simulink model "estTest"  (R2021b)
settings: Solver=FixedStepAuto  StartTime=0.0  StopTime=600  RelTol=1e-3
StartFcn:
  | hardwareSetup;
model workspace (MAT data in the model file):
  Ts = Simulink.Parameter
  Ts.Value = 0.005
  Ts.DataType = 'auto'
  Ts.Complexity = 'real'
  Ts.Dimensions = [1 1]
  stepH = Simulink.Parameter
  stepH.Value = 60
  stepH.DataType = 'auto'
  stepH.Complexity = 'real'
  stepH.Dimensions = [1 1]
  stepL = Simulink.Parameter
  stepL.Value = 50
  stepL.DataType = 'auto'
  stepL.Complexity = 'real'
  stepL.Dimensions = [1 1]
  tF = Simulink.Parameter
  tF.Value = 0.3
  tF.DataType = 'auto'
  tF.Complexity = 'real'
  tF.Dimensions = [1 1]
  tS = Simulink.Parameter
  tS.Value = 0.3
  tS.DataType = 'auto'
  tS.Complexity = 'real'
  tS.Dimensions = [1 1]
values from neighbouring files (symbols this model uses):
  Ts = 0.025    [MPCGen_OffsetFree.m]    (also in MPCGen_OffsetFree_UD.m = 0.02; MPCGen_OffsetFree_estDis.m = 0.03; MPCcontrollerGen_OffsetFree.m; MPCcontrollerGen_OffsetFree_UD.m = 0.02)
libraries: PuppyLibrary x6
settings Model: SimulationMode=external  ExtModeTrigDuration=2  Creator=kboxi  LastModifiedBy=MSI-NB
settings SolverCC: AlgebraicLoopSolver=TrustRegion  PositivePriorityOrder=on
settings DataIOCC: LimitDataPoints=on  MaxDataPoints=10000
settings OptimizationCC: DefaultParameterBehavior=Inlined  MaxStackSize=64
settings DebuggingCC: ParameterTunabilityLossMsg=error  SFMachineParentedDataDiag=warning  ArithmeticOperatorsInVariantConditions=warning
settings HardwareCC: ProdBitPerPointer=32  ProdBitPerSizeT=32  ProdBitPerPtrDiffT=32  ProdLargestAtomicInteger=Long  ProdLargestAtomicFloat=Double  ProdWordSize=32  ProdHWDeviceType=ARM Compatible->ARM Cortex  UseEmbeddedCoderFeatures=off
settings SFSimCC: SimUseLocalCustomCode=off  CustomCodeUndefinedFunction=UseInterfaceOnly
settings RTWCC: Description=Embedded Coder  SystemTargetFile=ert.tlc  HardwareBoard=Raspberry Pi  TLCOptions="-aInlineSetEventsForThisBaseRateFcn=TLC_FALSE -aSuppressMultiTaskScheduler=TLC_FALSE  -aRateBasedStepFcn=0"  TemplateMakefile=ert_default_tmf  RTWUseLocalCustomCode=off  Toolchain=GNU GCC Embedded Linux  BuildConfiguration=Faster Runs
settings CodeAppCC: ForceParamTrailComments=on  GenerateComments=off  OperatorAnnotations=on  StateflowObjectComments=on  MATLABSourceComments=on
settings ERTTargetCC: ERTCustomFileBanners=off  MatFileLogging=on  SupportContinuousTime=on  SupportNonInlinedSFcns=on  RemoveResetFunc=off  SupportVariableSizeSignals=on  ModelStepFunctionPrototypeControlCompliant=off  ExtModeTransport=2  ExtModeStaticAlloc=on  ExtModeMexFile=ext_xcp  ExtModeIntrfLevel=Level2 - Open

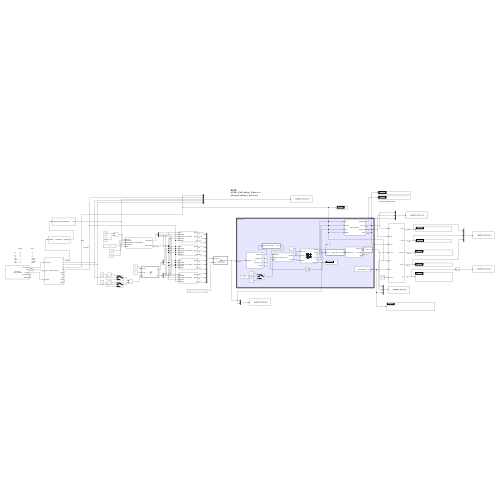
[thumbnail: Simulink's stored preview of the top-level diagram]
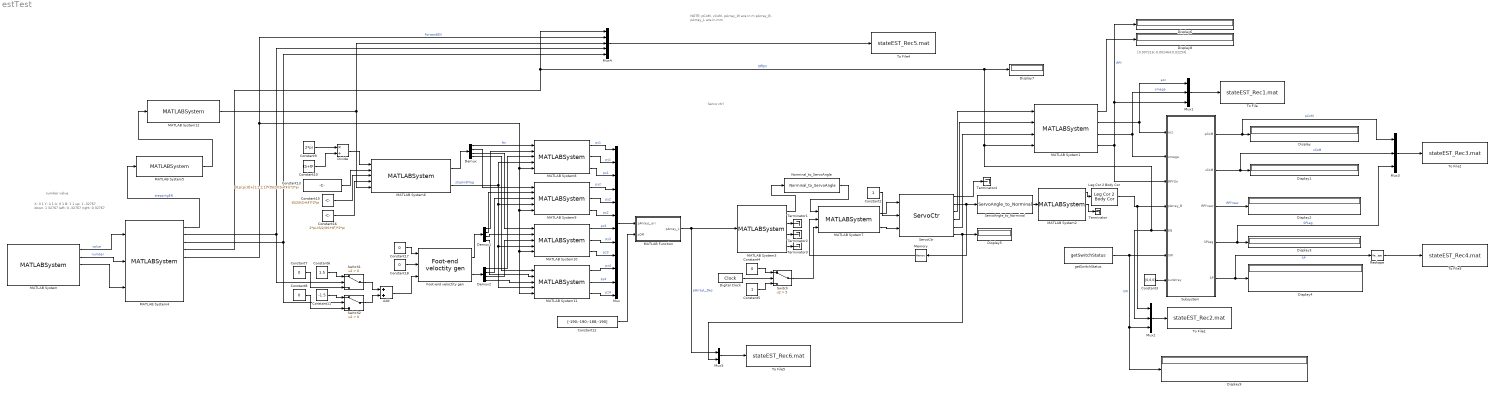
== system estTest ==
  note: NOTE:
      | pCoM, vCoM, pArray_W are in m
      | pArray_B, pArray_L are in mm
  note: Servo ctrl
  note: number value
  note: X:            3                                   1
      | Y:            4                                   1
      | A:            0                                   1
      | B:            1                                   1
      | up:           1                               -32767
      | down:      1                                32767
      | left:          0                                -32767
      | right:        0                               32767
  note: [0.007216;-0.002464;0.02254]
  Add : Sum
  Constant10 : Constant  Value=tS+tF
  Constant11 : Constant  Value=-1.5
  Constant12 : Constant  Value=[-190;-190;-188;-190]
  Constant13 : Constant  Value=[0;pi;pi;0]+[1;1;1;1]*(tS/2/(tS+tF))*2*pi
  Constant15 : Constant  Value=tS/2/(tS+tF)*2*pi
  Constant16 : Constant  Value=2*pi-tS/2/(tS+tF)*2*pi
  Constant{4,7..8,17..18} (5 alike) : Constant  Value=0
  Constant2 : Constant
  Constant3 : Constant  Value=[0,0,0]
  Constant5 : Constant
  Constant6 : Constant  Value=1.5
  Constant9 : Constant  Value=2*pi
  Demux : Demux
  Demux1 : Demux
  Demux2 : Demux
  Digital Clock : DigitalClock  SampleTime=Ts
  Display{,1..9} (10 alike) : Display
  Divide : Product  Inputs=*/
  Foot-end veloctity gen : PuppyLibrary/Foot-end veloctity gen  SystemSampleTime=-1  VariantActivationTime=update diagram  Latency=0  AutoFrameSizeCalculation=off
  Leg Cor 2 Body Cor : PuppyLibrary/Leg Cor 2 Body Cor  SystemSampleTime=-1  VariantActivationTime=update diagram  Latency=0  AutoFrameSizeCalculation=off
  MATLAB Function : MATLAB Function  TreatAsAtomicUnit=on
  MATLAB System : MATLABSystem  System=JoystickRead  SampleTime=0.005
      mask Type: JoystickRead
      mask Display:
      | disp(['Bluetooth' char(10) ' Joystick Reader']);
      | port_label('output',1,'EventNum');
      | port_label('output',2,'value');
      | port_label('output',3,'number');
      | port_label('output',4,'buttonState');
      | port_label('output',5,'axisState');
  MATLAB System1 : MATLABSystem  System=IMU_regulation  SimulateUsing=Code generation
      mask Type: IMU_regulation
      mask Display:
      | disp('IMU_regulation');
      | port_label('input',1,'acc');
      | port_label('input',2,'omega');
      | port_label('input',3,'rpy');
      | port_label('input',4,'OffEN');
      | port_label('output',1,'accOffnow');
      | port_label('output',2,'accL_W');
      | port_label('output',3,'omega_W');
      | port_label('output',4,'RPY');
  MATLAB System10 : MATLABSystem  System=cycCurveGen  Tf=tF  Ts=tS  H=stepH  L=stepL  Hsd=3  dt=Ts  SimulateUsing=Code generation
      mask Type: cycCurveGen
      mask Display:
      | disp('cycCurveGen');
      | port_label('input',1,'fai');
      | port_label('input',2,'vpxAdd');
      | port_label('input',3,'vpyAdd');
      | port_label('input',4,'stopInd');
      | port_label('input',5,'xADes');
      | port_label('output',1,'pxOut');
      | port_label('output',2,'pyOut');
      | port_label('output',3,'pz');
  MATLAB System11 : MATLABSystem  System=cycCurveGen  Tf=tF  Ts=tS  H=stepH  L=stepL  Hsd=4  dt=Ts  SimulateUsing=Code generation
      mask Type: cycCurveGen
      mask Display:
      | disp('cycCurveGen');
      | port_label('input',1,'fai');
      | port_label('input',2,'vpxAdd');
      | port_label('input',3,'vpyAdd');
      | port_label('input',4,'stopInd');
      | port_label('input',5,'xADes');
      | port_label('output',1,'pxOut');
      | port_label('output',2,'pyOut');
      | port_label('output',3,'pz');
  MATLAB System12 : MATLABSystem  System=ButtonHoldviaEdge  SimulateUsing=Code generation
      mask Type: ButtonHoldviaEdge
      mask Display:
      | disp('ButtonHoldviaEdge');
      | port_label('input',1,'dataEdge');
      | port_label('output',1,'data');
  MATLAB System2 : MATLABSystem  System=FK  dt=0.005  SimulateUsing=Code generation
      mask Type: FK
      mask Display:
      | disp('FK');
      | port_label('input',1,'AngleArray');
      | port_label('output',1,'pArray_L');
      | port_label('output',2,'errFlag');
      | port_label('output',3,'dq');
  MATLAB System3 : MATLABSystem  System=IK  LF_Off=[ 0; 0; 0 ]  RF_Off=[ 0; 0; 0 ]  LH_Off=[ 0; 0; 0 ]  RH_Off=[ 0; 0; 0 ]  SimulateUsing=Code generation
      mask Type: IK
      mask Display:
      | disp('IK');
      | port_label('input',1,'pArray_L');
      | port_label('output',1,'AngleArray');
      | port_label('output',2,'OffsetPArray');
      | port_label('output',3,'pArray_L_Out');
      | port_label('output',4,'errFlag');
  MATLAB System4 : MATLABSystem  System=buttonDecoder_2  SimulateUsing=Code generation
      mask Type: buttonDecoder_2
      mask Display:
      | disp('buttonDecoder_2');
      | port_label('input',1,'Eventnum');
      | port_label('input',2,'value');
      | port_label('input',3,'number');
      | port_label('output',1,'X');
      | port_label('output',2,'Y');
      | port_label('output',3,'A');
      | port_label('output',4,'B');
      | port_label('output',5,'up');
      | port_label('output',6,'down');
      | port_label('output',7,'left');
      | port_label('output',8,'right');
      | port_label('output',9,'LAxis');
      | port_label('output',10,'RAxis');
  MATLAB System5 : MATLABSystem  System=edgeDetector  SimulateUsing=Code generation
      mask Type: edgeDetector
      mask Display:
      | disp('edgeDetector');
      | port_label('input',1,'dataNow');
      | port_label('output',1,'dataEdge');
  MATLAB System6 : MATLABSystem  System=PhaseOscillator  SampleTime=Ts  OffsetTime=0  TickTime=0.1  SimulateUsing=Code generation
      mask Type: PhaseOscillator
      mask Display:
      | disp('PhaseOscillator');
      | port_label('input',1,'omega');
      | port_label('input',2,'phaseLag');
      | port_label('input',3,'stopIndPhase');
      | port_label('input',4,'stopPhase');
      | port_label('input',5,'EN');
      | port_label('output',1,'phaseNow');
      | port_label('output',2,'stopIndFlag');
  MATLAB System7 : MATLABSystem  System=PosAssign_vel  cons_Vel=15  dt=Ts  SimulateUsing=Code generation
      mask Type: PosAssign_vel
      mask Display:
      | disp('PosAssign_vel');
      | port_label('input',1,'PosDes');
      | port_label('input',2,'PosNow');
      | port_label('input',3,'EN');
      | port_label('output',1,'PosOut');
      | port_label('output',2,'setEN');
  MATLAB System8 : MATLABSystem  System=cycCurveGen  Tf=tF  Ts=tS  H=stepH  L=stepL  Hsd=4  dt=Ts  SimulateUsing=Code generation
      mask Type: cycCurveGen
      mask Display:
      | disp('cycCurveGen');
      | port_label('input',1,'fai');
      | port_label('input',2,'vpxAdd');
      | port_label('input',3,'vpyAdd');
      | port_label('input',4,'stopInd');
      | port_label('input',5,'xADes');
      | port_label('output',1,'pxOut');
      | port_label('output',2,'pyOut');
      | port_label('output',3,'pz');
  MATLAB System9 : MATLABSystem  System=cycCurveGen  Tf=tF  Ts=tS  H=stepH  L=stepL  Hsd=4  dt=Ts  SimulateUsing=Code generation
      mask Type: cycCurveGen
      mask Display:
      | disp('cycCurveGen');
      | port_label('input',1,'fai');
      | port_label('input',2,'vpxAdd');
      | port_label('input',3,'vpyAdd');
      | port_label('input',4,'stopInd');
      | port_label('input',5,'xADes');
      | port_label('output',1,'pxOut');
      | port_label('output',2,'pyOut');
      | port_label('output',3,'pz');
  Memory : Memory  InitialCondition=zeros(12,1)
  Mux : Mux  Inputs=12
  Mux1 : Mux  Inputs=3
  Mux2 : Mux  Inputs=3
  Mux3 : Mux  Inputs=3
  Mux4 : Mux  Inputs=5
  Mux5 : Mux  Inputs=2
  Norminal_to_ServoAngle : PuppyLibrary/Norminal_to_ServoAngle  SystemSampleTime=-1  VariantActivationTime=update diagram  Latency=0  AutoFrameSizeCalculation=off
  Reshape : Reshape
  ServoAngle_to_Norminal : PuppyLibrary/ServoAngle_to_Norminal  SystemSampleTime=-1  VariantActivationTime=update diagram  Latency=0  AutoFrameSizeCalculation=off
  ServoCtr : PuppyLibrary/ServoCtr  SystemSampleTime=-1  VariantActivationTime=update diagram  Latency=0  AutoFrameSizeCalculation=off
  Subsystem : Subsystem
  Switch : Switch  Criteria=u2 > Threshold  Threshold=5
  Switch1 : Switch  Criteria=u2 > Threshold
  Switch2 : Switch  Criteria=u2 > Threshold
  Terminator{,1..4} (5 alike) : Terminator
  To File : ToFile  Filename=stateEST_Rec1.mat  MatrixName=in_acc_omega_RPY
  To File1 : ToFile  Filename=stateEST_Rec2.mat  MatrixName=in_pArrayB_EN_SW
  To File2 : ToFile  Filename=stateEST_Rec3.mat  MatrixName=est_pCoM_vCoM_SPLeg
  To File3 : ToFile  Filename=stateEST_Rec4.mat  MatrixName=est_SP
  To File4 : ToFile  Filename=stateEST_Rec5.mat  MatrixName=est_offEN_forward_step_left_right
  To File5 : ToFile  Filename=stateEST_Rec6.mat  MatrixName=est_pArrayLDes_stm32Error
  getSwitchStatus : PuppyLibrary/getSwitchStatus  sampleTime=0.005
  wires:
  Reshape/1 -> To File3/1
  MATLAB System4/3 -> Switch2/2, Mux4/5
  MATLAB System4/4 -> Mux4/1, Mux2/2, Subsystem/5(EN), MATLAB System1/4, Display7/1  "OffEN"
  MATLAB System5/1 -> MATLAB System12/1
  Mux1/1 -> To File/1
  Mux2/1 -> To File1/1
  MATLAB System2/1 -> Leg Cor 2 Body Cor/1
  MATLAB System4/5 -> Mux4/2, MATLAB System8/5, MATLAB System11/5, MATLAB System10/5, MATLAB System9/5  "ForwardEN"
  MATLAB System2/2 -> Terminator/1
  MATLAB System1/3 -> Mux1/2, Subsystem/2(omega)  "omega"
  MATLAB System1/2 -> Subsystem/1(acc), Mux1/1  "acc"
  MATLAB System9/3 -> Mux/6  "pz2"
  MATLAB System1/4 -> Mux1/3, Display6/1, Subsystem/3(RPYOri)  "RPY"
  Demux1/1 -> MATLAB System8/2
  ServoCtr/4 -> MATLAB System1/2
  MATLAB System8/2 -> Mux/2  "py1"
  MATLAB System4/2 -> Switch1/2, Mux4/4
  Demux2/4 -> MATLAB System11/3
  MATLAB System3/3 -> Terminator2/1
  ServoCtr/1 -> Terminator4/1
  getSwitchStatus/1 -> Display9/1, Mux2/3, Subsystem/6(SW)  "SW"
  Memory/1 -> MATLAB System7/2
  MATLAB System6/2 -> MATLAB System11/4, MATLAB System10/4, MATLAB System9/4, MATLAB System8/4  "stopIndFlag"
  MATLAB System1/1 -> Display8/1
  Constant6/1 -> Switch1/1
  Switch2/1 -> Add/2
  Constant13/1 -> MATLAB System6/2
  Demux/2 -> MATLAB System9/1
  MATLAB System7/2 -> ServoCtr/3
  ServoCtr/6 -> Mux5/2, Display5/1
  ServoCtr/3 -> MATLAB System1/1
  MATLAB System11/3 -> Mux/12  "pz4"
  MATLAB Function/1(pArray_L) -> Mux5/1, MATLAB System3/1  "pArrayL_Des"
  ServoCtr/5 -> MATLAB System1/3
  MATLAB System8/1 -> Mux/1  "px1"
  MATLAB System/3 -> MATLAB System4/3
  Subsystem/5(SP) -> Reshape/1, Display4/1  "SP"
  Demux2/1 -> MATLAB System8/3
  Constant12/1 -> MATLAB Function/2(zOff)
  Mux/1 -> MATLAB Function/1(pArrayL_ori)
  Constant7/1 -> Switch1/3
  Demux/3 -> MATLAB System10/1
  Subsystem/1(pCoM) -> Mux3/1, Display/1  "pCoM"
  Switch1/1 -> Add/1
  MATLAB System11/2 -> Mux/11  "py4"
  Demux2/3 -> MATLAB System10/3
  Constant8/1 -> Switch2/3
  MATLAB System12/1 -> Mux4/3, MATLAB System6/5
  Demux1/4 -> MATLAB System11/2
  MATLAB System3/1 -> Norminal_to_ServoAngle/1
  MATLAB System10/3 -> Mux/9  "pz3"
  MATLAB System11/1 -> Mux/10  "px4"
  Add/1 -> Foot-end veloctity gen/3
  MATLAB System9/2 -> Mux/5  "py2"
  ServoCtr/2 -> Memory/1, ServoAngle_to_Norminal/1
  MATLAB System3/4 -> Terminator3/1
  Constant17/1 -> Foot-end veloctity gen/1
  Foot-end veloctity gen/1 -> Demux1/1
  Constant9/1 -> Divide/1
  Divide/1 -> MATLAB System6/1
  Foot-end veloctity gen/2 -> Demux2/1
  MATLAB System6/1 -> Demux/1
  Norminal_to_ServoAngle/1 -> MATLAB System7/1
  Constant16/1 -> MATLAB System6/4
  MATLAB System8/3 -> Mux/3  "pz1"
  Constant4/1 -> Switch/1
  Demux/4 -> MATLAB System11/1
  Digital Clock/1 -> Switch/2
  Constant15/1 -> MATLAB System6/3
  Demux1/2 -> MATLAB System9/2
  ServoAngle_to_Norminal/1 -> MATLAB System2/1
  Subsystem/4(SPLeg) -> Mux3/3, Display3/1  "SPLeg"
  MATLAB System10/2 -> Mux/8  "py3"
  Demux2/2 -> MATLAB System9/3
  Constant18/1 -> Foot-end veloctity gen/2
  Subsystem/3(RPYnew) -> Display2/1  "RPYnew"
  Constant5/1 -> Switch/3
  Constant3/1 -> Subsystem/7(surArray)
  MATLAB System4/1 -> MATLAB System5/1  "steppingEN"
  Constant2/1 -> ServoCtr/2
  Switch/1 -> MATLAB System7/3
  MATLAB System10/1 -> Mux/7  "px3"
  MATLAB System3/2 -> Terminator1/1
  Constant11/1 -> Switch2/1
  MATLAB System9/1 -> Mux/4  "px2"
  MATLAB System/2 -> MATLAB System4/2  "number"
  Demux/1 -> MATLAB System8/1  "fai"
  Leg Cor 2 Body Cor/1 -> Mux2/1, Subsystem/4(pArray_B)
  Demux1/3 -> MATLAB System10/2
  Mux3/1 -> To File2/1
  MATLAB System7/1 -> ServoCtr/1
  Subsystem/2(vCoM) -> Mux3/2, Display1/1  "vCoM"
  MATLAB System/1 -> MATLAB System4/1  "value"
  Constant10/1 -> Divide/2
  Mux4/1 -> To File4/1
  Mux5/1 -> To File5/1

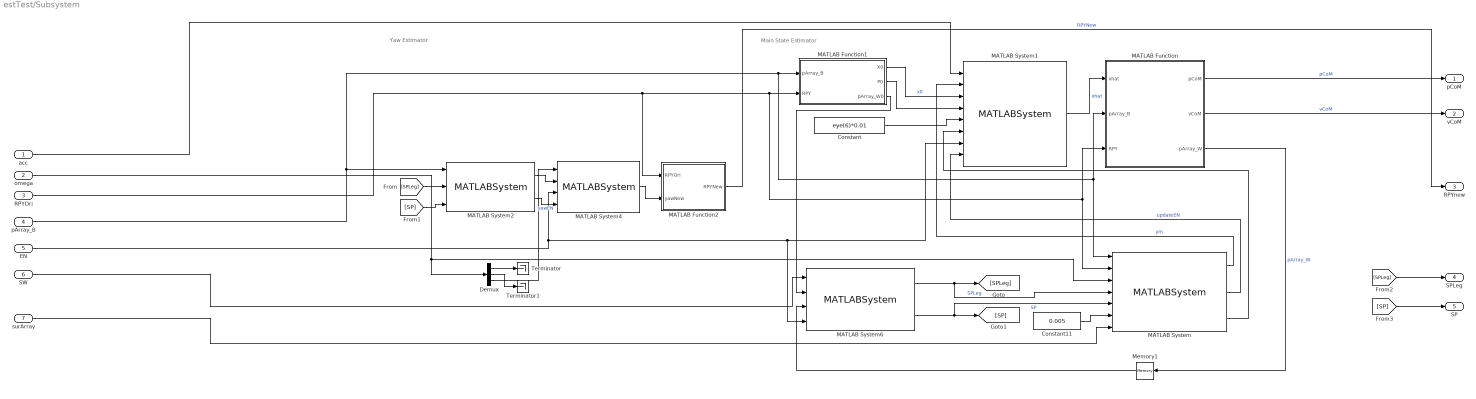
== system estTest/Subsystem ==
  note: Yaw Estimator
  note: Main State Estimator
  acc : Inport
  omega : Inport  Port=2
  RPYOri : Inport  Port=3
  pArray_B : Inport  Port=4
  EN : Inport  Port=5
  SW : Inport  Port=6
  surArray : Inport  Port=7
  Constant : Constant  Value=eye(6)*0.01
  Constant11 : Constant  Value=0.005
  Demux : Demux  Outputs=3
  MATLAB Function : MATLAB Function  TreatAsAtomicUnit=on
  MATLAB Function1 : MATLAB Function  TreatAsAtomicUnit=on
  MATLAB Function2 : MATLAB Function  TreatAsAtomicUnit=on
  MATLAB System : MATLABSystem  System=estX_byJoint  SimulateUsing=Code generation
      mask Type: estX_byJoint
      mask Display:
      | disp('estX_byJoint');
      | port_label('input',1,'pArray_B');
      | port_label('input',2,'RPY');
      | port_label('input',3,'omegaB');
      | port_label('input',4,'SPLeg');
      | port_label('input',5,'SP');
      | port_label('input',6,'dt');
      | port_label('input',7,'surPara');
      | port_label('output',1,'ym');
      | port_label('output',2,'updateEN');
      | port_label('output',3,'KF_R');
  MATLAB System1 : MATLABSystem  System=KalmanFilter_DIY  Ts=0.005  SimulateUsing=Code generation
      mask Type: KalmanFilter_DIY
      mask Display:
      | disp('KalmanFilter_DIY');
      | port_label('input',1,'u');
      | port_label('input',2,'y');
      | port_label('input',3,'x0');
      | port_label('input',4,'p0');
      | port_label('input',5,'Q');
      | port_label('input',6,'R');
      | port_label('input',7,'Reset');
      | port_label('input',8,'updateEN');
      | port_label('output',1,'xhat');
  MATLAB System2 : MATLABSystem  System=yawEst_byJoint  dt=0.005  SimulateUsing=Code generation
      mask Type: yawEst_byJoint
      mask Display:
      | disp('yawEst_byJoint');
      | port_label('input',1,'pArray_B');
      | port_label('input',2,'SPLeg');
      | port_label('input',3,'SP');
      | port_label('output',1,'yawKine');
      | port_label('output',2,'updateEN');
  MATLAB System4 : MATLABSystem  System=KalmanFilter_DIY_yaw  A=1  B=Ts  C=1  G=1  x0=0  p0=1  Q=0.1  R=0.1  SimulateUsing=Code generation
      mask Type: KalmanFilter_DIY_yaw
      mask Display:
      | disp('KalmanFilter_DIY_yaw');
      | port_label('input',1,'u');
      | port_label('input',2,'y');
      | port_label('input',3,'Reset');
      | port_label('input',4,'updateEN');
      | port_label('output',1,'xhat');
  MATLAB System6 : MATLABSystem  System=LegStateIndicator  SimulateUsing=Code generation
      mask Type: LegStateIndicator
      mask Display:
      | disp('LegStateIndicator');
      | port_label('input',1,'SW');
      | port_label('input',2,'pArray_W0');
      | port_label('input',3,'pArray_W');
      | port_label('input',4,'reset');
      | port_label('output',1,'SPLeg');
      | port_label('output',2,'SP');
  Memory1 : Memory  InitialCondition=zeros(12,1)  InheritSampleTime=on
  Terminator : Terminator
  Terminator1 : Terminator
  pCoM : Outport
  vCoM : Outport  Port=2
  RPYnew : Outport  Port=3
  SPLeg : Outport  Port=4
  SP : Outport  Port=5
  wires:
  Demux/1 -> Terminator/1
  MATLAB System6/2 -> [SP], MATLAB System/5  "SP"
  MATLAB System/1 -> MATLAB System1/2  "ym"
  MATLAB System/2 -> MATLAB System1/8  "updateEN"
  Demux/3 -> MATLAB System4/1
  [SPLeg] -> MATLAB System2/2
  Constant/1 -> MATLAB System1/5
  MATLAB System4/1 -> MATLAB Function2/2(yawNew)
  MATLAB System2/1 -> MATLAB System4/2
  MATLAB System1/1 -> MATLAB Function/1(xhat)  "xhat"
  pArray_B/1 -> MATLAB System2/1, MATLAB Function1/1(pArray_B), MATLAB Function/2(pArray_B), MATLAB System/1
  MATLAB Function1/1(X0) -> MATLAB System1/3  "x0"
  MATLAB Function/1(pCoM) -> pCoM/1  "pCoM"
  MATLAB System/3 -> MATLAB System1/6
  MATLAB System6/1 -> MATLAB System/4, [SPLeg]  "SPLeg"
  MATLAB Function1/3(pArray_W0) -> MATLAB System6/2
  Demux/2 -> Terminator1/1
  RPYOri/1 -> MATLAB Function2/1(RPYOri), MATLAB Function1/2(RPY), MATLAB Function/3(RPY), MATLAB System/2
  MATLAB Function/2(vCoM) -> vCoM/1  "vCoM"
  EN/1 -> MATLAB System4/3, MATLAB System1/7, MATLAB System6/4
  Constant11/1 -> MATLAB System/6
  MATLAB Function1/2(P0) -> MATLAB System1/4
  surArray/1 -> MATLAB System/7
  MATLAB Function/3(pArray_W) -> Memory1/1  "pArray_W"
  omega/1 -> Demux/1, MATLAB System/3
  MATLAB System2/2 -> MATLAB System4/4  "yawEN"
  [SP] -> MATLAB System2/3
  Memory1/1 -> MATLAB System6/3
  [SPLeg] -> SPLeg/1
  [SP] -> SP/1
  acc/1 -> MATLAB System1/1
  SW/1 -> MATLAB System6/1
  MATLAB Function2/1(RPYNew) -> RPYnew/1  "RPYNew"

== matlab function estTest/Subsystem/MATLAB Function1 ==
  data: pArray_B input; RPY input; X0 output; P0 output; pArray_W0 output
function [X0,P0,pArray_W0]=fcn(pArray_B,RPY)
% NOTE: pArray_W0 is calculated without the value of yaw angle!!!
Ry=[cos(RPY(2)),0,sin(RPY(2));
    0,1,0;
    -sin(RPY(2)),0,cos(RPY(2))];
Rx=[1,0,0;
    0,cos(RPY(1)),-sin(RPY(1));
    0,sin(RPY(1)),cos(RPY(1))];
pArray_B=reshape(pArray_B,3,4)/1000;
pArray_float=Ry*Rx*pArray_B; % foot-end position in floating coordinate
zOff=-min(pArray_float(3,:));
temp=pArray_float+[0;0;zOff]*[1,1,1,1];
pCoM=[0;0;zOff];
vCoM=[0;0;0];
pArray_W0=[temp(:,1);temp(:,2);temp(:,3);temp(:,4)];
X0=[pCoM;vCoM];
P0=eye(6);

== matlab function estTest/Subsystem/MATLAB Function ==
  data: xhat input size=[6,1]; pCoM output size=[3,1]; vCoM output size=[3,1]; pArray_B input; RPY input; pArray_W output
function [pCoM,vCoM,pArray_W] = fcn(xhat,pArray_B,RPY)
% pB the CoM position in the world coordinate
% vB the CoM velocity
% Wpi the foot-end position in the world coordinate
pCoM=[xhat(1);xhat(2);xhat(3)];
vCoM=[xhat(4);xhat(5);xhat(6)];
Rz=[cos(RPY(3)),-sin(RPY(3)),0;
    sin(RPY(3)),cos(RPY(3)),0;
    0,0,1];
Ry=[cos(RPY(2)),0,sin(RPY(2));
    0,1,0;
    -sin(RPY(2)),0,cos(RPY(2))];
Rx=[1,0,0;
    0,cos(RPY(1)),-sin(RPY(1));
    0,sin(RPY(1)),cos(RPY(1))];
R=Rz*Ry*Rx;
pArray_B=reshape(pArray_B,3,4)/1000;
temp=R*pArray_B+pCoM*[1,1,1,1];
pArray_W=[temp(:,1);temp(:,2);temp(:,3);temp(:,4)];

== matlab function estTest/Subsystem/MATLAB Function2 ==
  data: RPYOri input; RPYNew output size=[3 1]; yawNew input
function RPYNew = fcn(RPYOri,yawNew)
RPYNew=zeros(3,1);
RPYNew(1)=RPYOri(1);
RPYNew(2)=RPYOri(2);
RPYNew(3)=yawNew;

== matlab function estTest/MATLAB Function ==
  data: pArrayL_ori input; pArray_L output; zOff input
function pArray_L = footEndOffset(pArrayL_ori,zOff)
pArray_L=pArrayL_ori+[0;37;zOff(1);0;-37;zOff(2);0;37;zOff(3);0;-37;zOff(4)];
